simulink model "CartPend_OL"  (R2023b)
settings: Solver=FixedStepDiscrete  StartTime=0.0  StopTime=10.0  FixedStep=0.001  RelTol=1e-3  EnableMultiTasking=on
values from neighbouring files (symbols this model uses):
  Ts = 0.01    [main.m]
undefined symbols (not defined in the file or in its folder): CEcosimulation, CoSimulate1
libraries: instrumentlib x2, cstblocks x2
settings Model: Creator=Aleksandr Prokhorov  LastModifiedBy=Aleksandr Prokhorov
settings SolverCC: AutoInsertRateTranBlk=on
settings DataIOCC: SaveOutput=off  SaveTime=off
settings OptimizationCC: DefaultParameterBehavior=Inlined  InlineInvariantSignals=on  EnhancedBackFolding=on  PassReuseOutputArgsAs=Individual arguments  StateBitsets=on  DataBitsets=on  ZeroExternalMemoryAtStartup=off  ZeroInternalMemoryAtStartup=off  NoFixptDivByZeroProtection=on  LifeSpan=1  OptimizeBlockOrder=speed  DifferentSizesBufferReuse=on  EfficientTunableParamExpr=on
settings DebuggingCC: ParameterTunabilityLossMsg=error
settings HardwareCC: ProdBitPerPointer=32  ProdBitPerSizeT=32  ProdBitPerPtrDiffT=32  ProdLargestAtomicFloat=None  ProdIntDivRoundTo=Floor  ProdWordSize=32  ProdHWDeviceType=Generic->Custom
settings SFSimCC: MATLABDynamicMemAlloc=off
settings RTWCC: Description=Embedded Coder  SystemTargetFile=ert.tlc  TLCOptions=-p0  GenCodeOnly=on  TemplateMakefile=ert_default_tmf  GenerateReport=on  RTWVerbose=off  IncludeHyperlinkInReport=on  LaunchReport=on
settings CodeAppCC: ForceParamTrailComments=on  IgnoreCustomStorageClasses=off  OperatorAnnotations=on  SimulinkDataObjDesc=on  SFDataObjDesc=on  CustomSymbolStrGlobalVar=rt$N$M  CustomSymbolStrType=$N$M  CustomSymbolStrFcn=$N$M$F  CustomSymbolStrMacro=$N$M  InsertBlockDesc=on
settings ERTTargetCC: TargetLangStandard=C99 (ISO)  CodeReplacementLibrary=ISO_C  GenerateSampleERTMain=on  IncludeMdlTerminateFcn=off  SuppressErrorStatus=on  SupportAbsoluteTime=off  PurelyIntegerCode=on  SupportNonFinite=off  SupportComplex=off  InlinedParameterPlacement=NonHierarchical  RootIOFormat=Structure reference  ERTCustomFileTemplate=example_file_process.tlc

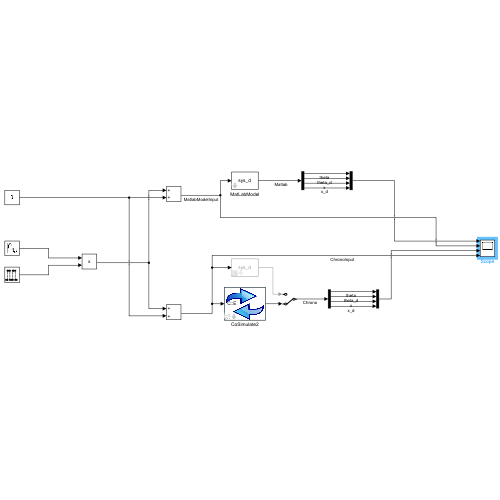
[thumbnail: Simulink's stored preview of the top-level diagram]
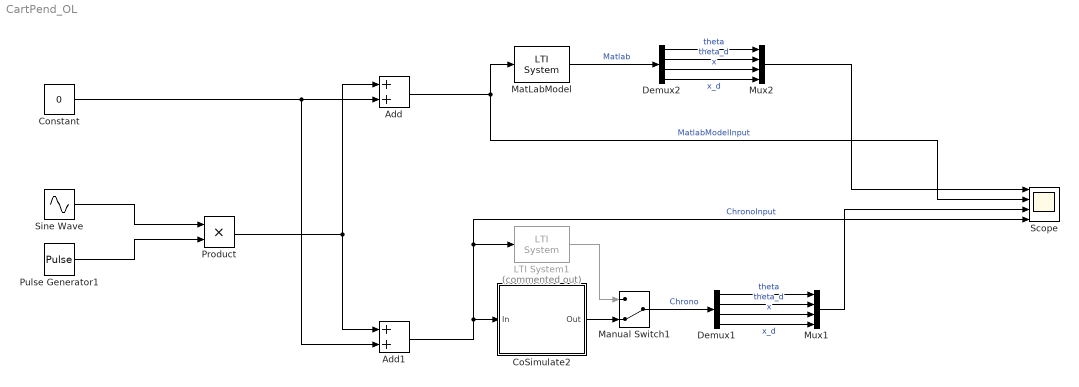
== system CartPend_OL ==
  Add : Sum
  Add1 : Sum
  CoSimulate2 : Subsystem  Description=|  Priority=100  AncestorBlock=CEcosimulation/CoSimulate1  mask{com_step=Ts, tcp_data_size=4, host_name=localhost, tcp_port=50009, tcp_timeout=15}
      | This block can be used to exchange data with Chrono::Engine.                                                                                      
      | A Chrono::Engine program with a running ChCosimulation inferface must be started, it will work as a server; then the Simulink program must be run.
      | Note! check that the dimensions of the exchanged vectors do match!
      mask prompts: com_step "Communication step size"; tcp_data_size "N. of scalars received from C::E (as block output)"; host_name "TCP host name (ex. 'localhost', or 'www.myhost.com')"; tcp_port "TCP port (ex. 50007)"; tcp_timeout "TCP timeout (seconds)"
      mask init:
      | block_receive = [gcb, '/TCP Receive'];
      | set_param(block_receive, 'SampleTime', num2str(com_step));
      | set_param(block_receive, 'Host', host_name);
      | set_param(block_receive, 'Port', num2str(tcp_port));
      | set_param(block_receive, 'DataSize', num2str(tcp_data_size+1));
      | set_param(block_receive, 'Timeout', num2str(tcp_timeout));
      | block_send = [gcb, '/TCP Send'];
      | set_param(block_send, 'Host', host_name);
      | set_param(block_send, 'Port', num2str(tcp_port));
      mask Display:
      | image(imread('block_logo.png'))
      | disp('C::E                   ')
  Constant : Constant  Value=0  SampleTime=Ts
  Demux1 : Demux
  Demux2 : Demux
  LTI System1 : cstblocks/LTI System  Commented=on  sys=sys_d  IC=[]  PadeOrder=0
  Manual Switch1 : ManualSwitch  CurrentSetting=0
  MatLabModel : cstblocks/LTI System  sys=sys_d  IC=[]  PadeOrder=0
  Mux1 : Mux
  Mux2 : Mux
  Product : Product
  Pulse Generator1 : DiscretePulseGenerator  Amplitude=0.01  Period=10/Ts  PulseWidth=0.05/Ts  PhaseDelay=1/Ts  SampleTime=Ts
  Scope : Scope  NumInputPorts=4
  Sine Wave : Sin  Amplitude=3e4  Frequency=50  Phase=0.35  SampleTime=Ts
  wires:
  Constant/1 -> Add1/2, Add/2
  Add/1 -> Scope/2, MatLabModel/1  "MatlabModelInput"
  Manual Switch1/1 -> Demux1/1  "Chrono"
  Mux1/1 -> Scope/3
  Demux1/1 -> Mux1/1  "theta"
  Demux1/4 -> Mux1/4  "x_d"
  Demux1/2 -> Mux1/2  "theta_d"
  Add1/1 -> Scope/4, LTI System1/1, CoSimulate2/1(In)  "ChronoInput"
  Demux1/3 -> Mux1/3  "x"
  Pulse Generator1/1 -> Product/2
  Sine Wave/1 -> Product/1
  Product/1 -> Add1/1, Add/1
  LTI System1/1 -> Manual Switch1/1
  CoSimulate2/1(Out) -> Manual Switch1/2
  Demux2/1 -> Mux2/1  "theta"
  Demux2/4 -> Mux2/4  "x_d"
  Demux2/3 -> Mux2/3  "x"
  MatLabModel/1 -> Demux2/1  "Matlab"
  Demux2/2 -> Mux2/2  "theta_d"
  Mux2/1 -> Scope/1

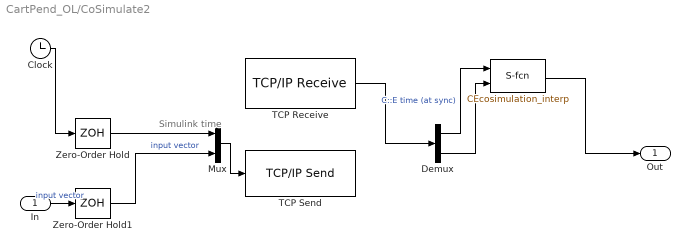
== system CartPend_OL/CoSimulate2 ==
  note: Simulink time
  In : Inport
  " " : M-S-Function  FunctionName=CEcosimulation_interp
  Clock : Clock
  Demux : Demux  Outputs=[1 -1]
  Mux : Mux  Inputs=2
  TCP Receive : instrumentlib/TCP//IP Receive  Priority=1  Host=localhost  Port=50009  DataSize=5  DataType=double  ASCIIFormatting=%f  Terminator=LF  CustomTerminator=10  ByteOrder=little-endian  EnableBlockingMode=on  Timeout=15  SampleTime=0.001  SimulateUsing=Interpreted execution
  TCP Send : instrumentlib/TCP//IP Send  Priority=2  Host=localhost  Port=50009  ByteOrder=little-endian  EnableBlockingMode=on  Timeout=10  TransferDelay=on  SimulateUsing=Interpreted execution
  Zero-Order Hold : ZeroOrderHold  Priority=0  SampleTime=com_step
  Zero-Order Hold1 : ZeroOrderHold  Priority=0  SampleTime=com_step
  Out : Outport
  wires:
  " "/1 -> Out/1
  Demux/2 -> " "/2
  Demux/1 -> " "/1  "C::E time (at sync)"
  Zero-Order Hold/1 -> Mux/1
  Zero-Order Hold1/1 -> Mux/2  "input vector"
  Mux/1 -> TCP Send/1
  Clock/1 -> Zero-Order Hold/1
  In/1 -> Zero-Order Hold1/1  "input vector"
  TCP Receive/1 -> Demux/1
